simulink model "Furuta_Template"  (Simulink 9.2)
settings: Solver=VariableStepAuto  StartTime=0.0  StopTime=50  FixedStep=0.001  RelTol=1e-8  EnableMultiTasking=on
values from neighbouring files (symbols this model uses):
  A = [0 0 1 0;0 0 0 1;0 LIN1 LIN2 LIN3;0 LIN4 LIN5 LIN6]    [changeable_parameters.m]
  A1 = -J2_hat*b1    (= -5.5028e-07)    [changeable_parameters.m]
  A2 = m2*L1*l2*b2    (= 8.64024e-07)    [changeable_parameters.m]
  A3 = -(J2_hat)^2    (= -3.028080784e-05)    [changeable_parameters.m]
  A4 = -(0.5)*J2_hat*m2*L1*l2    (= -8.49027012e-06)    [changeable_parameters.m]
  A5 = J2_hat*m2*L1*l2    (= 1.698054024e-05)    [changeable_parameters.m]
  A6 = J2_hat    (= 0.0055028)    [changeable_parameters.m]
  A7 = -m2*L1*l2    (= -0.0030858)    [changeable_parameters.m]
  A8 = 0.5*(m2^2)*(l2^2)*L1    (= 1.712619e-05)    [changeable_parameters.m]
  B1 = m2*L1*l2*b1    (= 3.0858e-07)    [changeable_parameters.m]
  B10 = J2_hat    (= 0.0055028)    [changeable_parameters.m]
  B11 = -m2*l2*J0_hat    (= -0.00014201673)    [changeable_parameters.m]
  B12 = -m2*l2*J2_hat    (= -6.108108e-05)    [changeable_parameters.m]
  B2 = -b2*J0_hat    (= -3.582404e-06)    [changeable_parameters.m]
  B3 = -b2*J2_hat    (= -1.540784e-06)    [changeable_parameters.m]
  B4 = m2*L1*l2*J2_hat    (= 1.698054024e-05)    [changeable_parameters.m]
  B5 = 0.5*J0_hat*J2_hat    (= 3.520223702e-05)    [changeable_parameters.m]
  B6 = 0.5*(J2_hat^2)    (= 1.514040392e-05)    [changeable_parameters.m]
  B7 = -0.5*(m2^2)*(L1^2)*(l2^2)    (= -4.76108082e-06)    [changeable_parameters.m]
  B8 = -m2*L1*l2    (= -0.0030858)    [changeable_parameters.m]
  B9 = J0_hat    (= 0.0127943)    [changeable_parameters.m]
  B_mod = [0;0;LIN7;LIN9]    [changeable_parameters.m]
  C = [1 0 0 0 ; 0 1 0 0 ]    [changeable_parameters.m]
  controller_gain_F = - lqr(A,B_mod,Q,R)    [changeable_parameters.m]
  D1 = J0_hat*J2_hat    (= 7.040447404e-05)    [changeable_parameters.m]
  D2 = J2_hat^2    (= 3.028080784e-05)    [changeable_parameters.m]
  D3 = -(m2^2)*(L1^2)*(l2^2)    (= -9.52216164e-06)    [changeable_parameters.m]
  E0 = 0    [changeable_parameters.m]
  G = 9.8    [changeable_parameters.m]
  J2_hat = J2+(m2*(l2^2))    (= 0.0055028)    [changeable_parameters.m]
  K_swingup = 10    [changeable_parameters.m]
  Km = 0.09    [SystemParameters.m]    (also in changeable_parameters.m)
  L = 0.005    [SystemParameters.m]    (also in changeable_parameters.m)
  l2 = 0.148    [SystemParameters.m]    (also in changeable_parameters.m)
  m2 = 0.075    [changeable_parameters.m]
  observer_gain_L = -place (A',C',obs_poles)'    [changeable_parameters.m]
  R = 7.8    [SystemParameters.m]    (also in changeable_parameters.m = B_mod'*Rh*Rh*B_mod)
libraries: simulink x1
settings Model: Creator=mecmg  LastModifiedBy=shady
settings OptimizationCC: ExpressionDepthLimit=2147483647
settings DebuggingCC: SolverPrmCheckMsg=warning

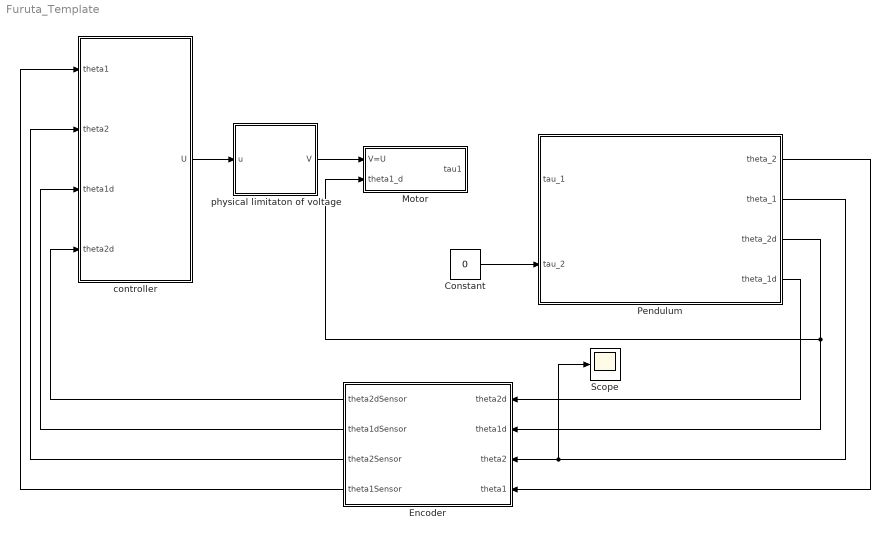
== system Furuta_Template ==
  Constant : Constant  Value=0  VectorParams1D=off
  Encoder : Subsystem
  Motor : Subsystem
  Pendulum : Subsystem
  Scope : Scope
  controller : Subsystem
  physical limitaton of voltage : Subsystem
  wires:
  Pendulum/4(theta_1d) -> Encoder/1(theta2d)
  Pendulum/3(theta_2d) -> Encoder/2(theta1d), Motor/2(theta1_d)
  Pendulum/2(theta_1) -> Scope/1, Encoder/3(theta2)
  Pendulum/1(theta_2) -> Encoder/4(theta1)
  physical limitaton of voltage/1(V) -> Motor/1(V=U)
  Encoder/1(theta2dSensor) -> controller/4(theta2d)
  Encoder/4(theta1Sensor) -> controller/1(theta1)
  Encoder/2(theta1dSensor) -> controller/3(theta1d)
  Encoder/3(theta2Sensor) -> controller/2(theta2)
  Constant/1 -> Pendulum/2(tau_2)
  controller/1("U ") -> physical limitaton of voltage/1(u)

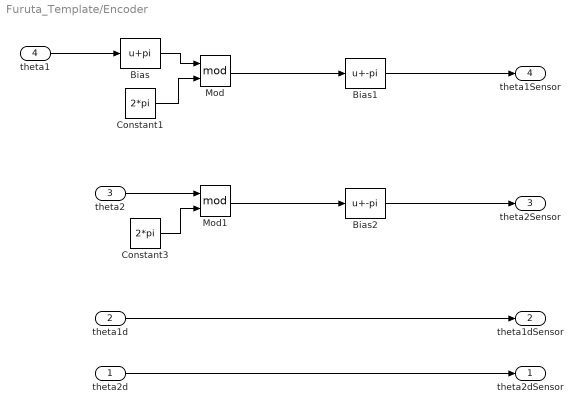
== system Furuta_Template/Encoder ==
  theta2d : Inport
  theta1d : Inport  Port=2
  theta2 : Inport  Port=3
  theta1 : Inport  Port=4
  Bias : Bias  Bias=pi
  Bias1 : Bias  Bias=-pi
  Bias2 : Bias  Bias=-pi
  Constant1 : Constant  Value=2*pi
  Constant3 : Constant  Value=2*pi
  Mod : Math  Operator=mod  SaturateOnIntegerOverflow=on
  Mod1 : Math  Operator=mod  SaturateOnIntegerOverflow=on
  theta2dSensor : Outport
  theta1dSensor : Outport  Port=2
  theta2Sensor : Outport  Port=3
  theta1Sensor : Outport  Port=4
  wires:
  theta1d/1 -> theta1dSensor/1
  theta2d/1 -> theta2dSensor/1
  theta1/1 -> Bias/1
  Constant1/1 -> Mod/2
  theta2/1 -> Mod1/1
  Constant3/1 -> Mod1/2
  Mod1/1 -> Bias2/1
  Bias/1 -> Mod/1
  Mod/1 -> Bias1/1
  Bias1/1 -> theta1Sensor/1
  Bias2/1 -> theta2Sensor/1

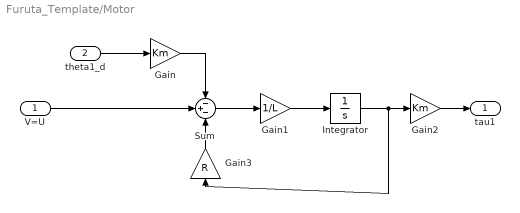
== system Furuta_Template/Motor ==
  V=U : Inport
  theta1_d : Inport  Port=2
  Gain : Gain  Gain=Km
  Gain1 : Gain  Gain=1/L
  Gain2 : Gain  Gain=Km
  Gain3 : Gain  Gain=R
  Integrator : Integrator
  Sum : Sum  Inputs=-+-
  tau1 : Outport
  wires:
  V=U/1 -> Sum/2
  Gain/1 -> Sum/1
  theta1_d/1 -> Gain/1
  Sum/1 -> Gain1/1
  Gain1/1 -> Integrator/1
  Integrator/1 -> Gain3/1, Gain2/1
  Gain2/1 -> tau1/1
  Gain3/1 -> Sum/3

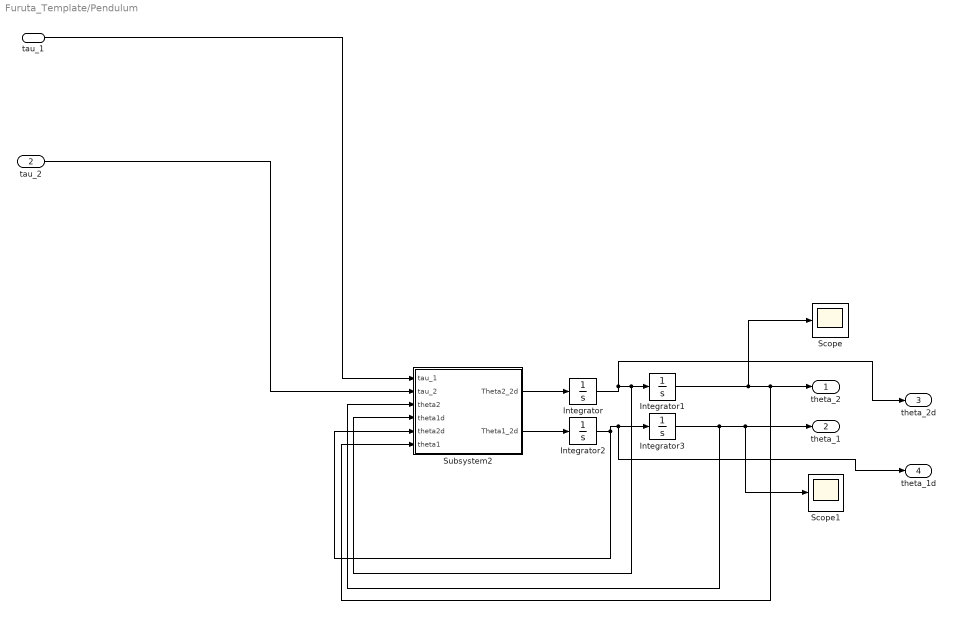
== system Furuta_Template/Pendulum ==
  "tau_1 " : Inport
  tau_2 : Inport  Port=2
  Integrator : Integrator
  Integrator1 : Integrator  InitialCondition=1
  Integrator2 : Integrator
  Integrator3 : Integrator  InitialCondition=1
  Scope : Scope
  Scope1 : Scope
  Subsystem2 : Subsystem
  theta_2 : Outport
  theta_1 : Outport  Port=2
  theta_2d : Outport  Port=3
  theta_1d : Outport  Port=4
  wires:
  tau_2/1 -> Subsystem2/2(tau_2)
  Integrator/1 -> theta_2d/1, Subsystem2/4(theta1d), Integrator1/1
  Integrator3/1 -> Subsystem2/3("theta2 "), Scope1/1, theta_1/1
  Integrator2/1 -> theta_1d/1, Integrator3/1, Subsystem2/5(theta2d)
  "tau_1 "/1 -> Subsystem2/1("tau_1 ")
  Integrator1/1 -> Scope/1, Subsystem2/6(theta1), theta_2/1
  Subsystem2/1(Theta2_2d) -> Integrator/1
  Subsystem2/2(Theta1_2d) -> Integrator2/1

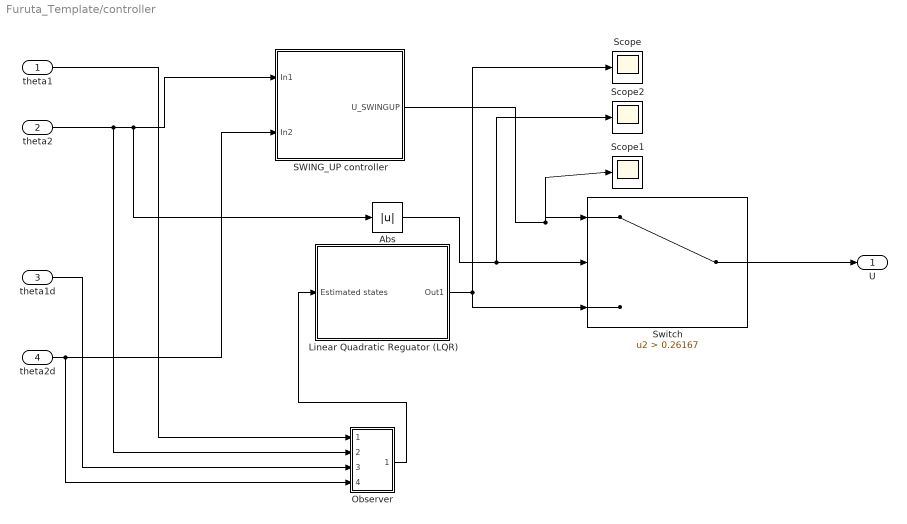
== system Furuta_Template/controller ==
  theta1 : Inport
  theta2 : Inport  Port=2
  theta1d : Inport  Port=3
  theta2d : Inport  Port=4
  " Linear Quadratic Reguator (LQR) " : Subsystem
  " Observer " : Subsystem
  " SWING_UP controller" : Subsystem
  Abs : Abs
  Scope : Scope
  Scope1 : Scope
  Scope2 : Scope
  Switch : Switch  Criteria=u2 > Threshold  Threshold=0.26167
  "U " : Outport
  wires:
  theta2/1 -> " Observer "/2(In3), Abs/1, " SWING_UP controller"/1(In1)
  theta2d/1 -> " Observer "/4(In5), " SWING_UP controller"/2(In2)
  " SWING_UP controller"/1(U_SWINGUP) -> Scope1/1, Switch/1
  Abs/1 -> Scope2/1, Switch/2
  Switch/1 -> "U "/1
  theta1/1 -> " Observer "/1(In1)
  theta1d/1 -> " Observer "/3(In4)
  " Linear Quadratic Reguator (LQR) "/1(Out1) -> Switch/3, Scope/1
  " Observer "/1(Estimated states) -> " Linear Quadratic Reguator (LQR) "/1("Estimated states ")

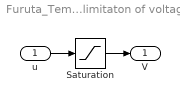
== system Furuta_Template/physical limitaton of voltage ==
  u : Inport
  Saturation : Saturate  UpperLimit=10  LowerLimit=-10
  V : Outport
  wires:
  u/1 -> Saturation/1
  Saturation/1 -> V/1

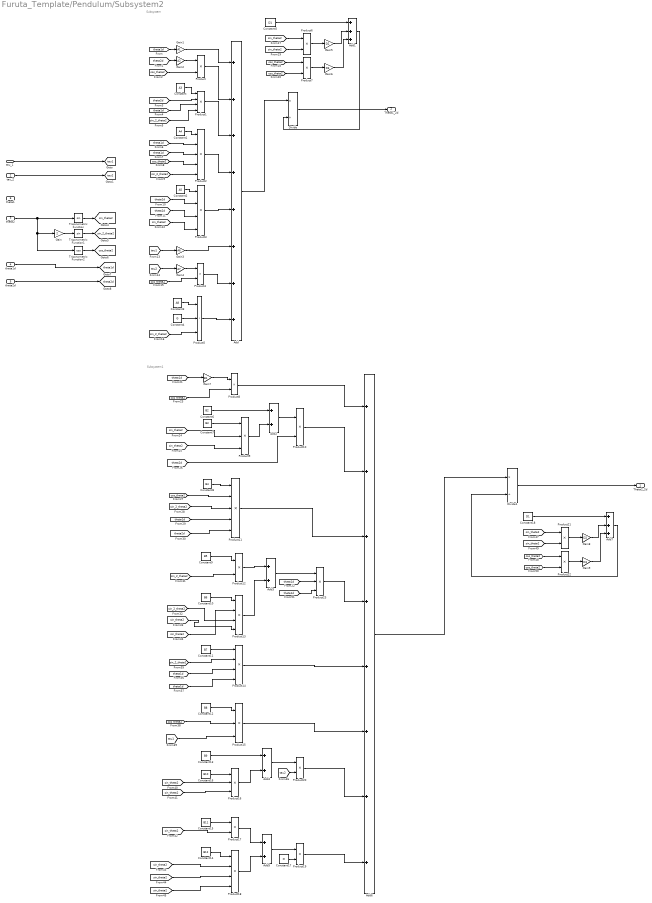
== system Furuta_Template/Pendulum/Subsystem2 ==
  note: Subsystem1
  note: Subsystem
  "tau_1 " : Inport
  tau_2 : Inport  Port=2
  "theta2 " : Inport  Port=3
  theta1d : Inport  Port=4
  theta2d : Inport  Port=5
  theta1 : Inport  Port=6
  Add : Sum  Inputs=8
  Add1 : Sum  Inputs=3
  Add{2..5} (4 alike) : Sum  Inputs=2
  Add6 : Sum  Inputs=8
  Add7 : Sum  Inputs=3
  Constant : Constant  Value=A3  VectorParams1D=off
  Constant1 : Constant  Value=A4  VectorParams1D=off
  Constant10 : Constant  Value=B6
  Constant11 : Constant  Value=B7
  Constant12 : Constant  Value=B8
  Constant13 : Constant  Value=B9
  Constant14 : Constant  Value=B12
  Constant15 : Constant  Value=B11
  Constant16 : Constant  Value=B10
  Constant17 : Constant  Value=G
  Constant18 : Constant  Value=D1
  Constant2 : Constant  Value=A5  VectorParams1D=off
  Constant3 : Constant  Value=A8  VectorParams1D=off
  Constant4 : Constant  Value=G  VectorParams1D=off
  Constant5 : Constant  Value=D1
  Constant6 : Constant  Value=B2
  Constant7 : Constant  Value=B3
  Constant8 : Constant  Value=B4
  Constant9 : Constant  Value=B5
  Divide : Product  Inputs=*/
  Divide1 : Product  Inputs=*/
  Gain : Gain  Gain=2
  Gain1 : Gain  Gain=A1
  Gain2 : Gain  Gain=A2
  Gain3 : Gain  Gain=A6
  Gain4 : Gain  Gain=A7
  Gain5 : Gain  Gain=D2
  Gain6 : Gain  Gain=D3
  Gain7 : Gain  Gain=B1
  Gain8 : Gain  Gain=D2
  Gain9 : Gain  Gain=D3
  Product{,6..7,21..22} (5 alike) : Product  OutMin=2
  Product{1,3,13..14,18} (5 alike) : Product  Inputs=4
  Product{4,8,10,12,17,19..20} (7 alike) : Product
  Product11 : Product  Inputs=5
  Product{5,9,15..16,23} (5 alike) : Product  Inputs=3
  Product2 : Product  Inputs=5
  Trigonometric Function : Trigonometry
  Trigonometric Function1 : Trigonometry
  Trigonometric Function2 : Trigonometry  Operator=cos
  Theta2_2d : Outport
  Theta1_2d : Outport  Port=2
  tag scope: cos_theta2=global, sin_2_theta2=global, sin_theta2=global, tau1=global, tau2=global, theta1d=global, theta2d=global
  wires:
  "theta2 "/1 -> Trigonometric Function2/1, Gain/1, Trigonometric Function/1
  Trigonometric Function1/1 -> [sin_2_theta2]
  theta2d/1 -> [theta2d]
  Trigonometric Function/1 -> [sin_theta2]
  Trigonometric Function2/1 -> [cos_theta2]
  tau_2/1 -> [tau2]
  "tau_1 "/1 -> [tau1]
  theta1d/1 -> [theta1d]
  Gain/1 -> Trigonometric Function1/1
  [theta2d] -> Product1/2
  Gain3/1 -> Add/6
  [sin_theta2] -> Product6/2
  [cos_theta2] -> Product7/2
  [sin_2_theta2] -> Product5/3
  Gain4/1 -> Product4/1
  Add1/1 -> Divide/2
  Product7/1 -> Gain6/1
  Gain1/1 -> Add/1
  [tau2] -> Gain4/1
  Constant1/1 -> Product2/1
  Product6/1 -> Gain5/1
  [cos_theta2] -> Product4/2
  [sin_2_theta2] -> Product2/5
  Product3/1 -> Add/5
  Gain5/1 -> Add1/2
  [theta2d] -> Product3/3
  Constant5/1 -> Add1/1
  [cos_theta2] -> Product7/1
  Gain2/1 -> Product/1
  [theta2d] -> Product3/2
  Product5/1 -> Add/8
  Product1/1 -> Add/3
  Product2/1 -> Add/4
  Gain6/1 -> Add1/3
  [theta1d] -> Product2/3
  [sin_theta2] -> Product3/4
  [cos_theta2] -> Product2/4
  [sin_theta2] -> Product6/1
  [theta1d] -> Product1/3
  Constant/1 -> Product1/1
  [theta1d] -> Product2/2
  [theta2d] -> Gain2/1
  [theta1d] -> Gain1/1
  Add/1 -> Divide/1
  [tau1] -> Gain3/1
  Product4/1 -> Add/7
  Constant4/1 -> Product5/2
  Product/1 -> Add/2
  [cos_theta2] -> Product/2
  Constant2/1 -> Product3/1
  [sin_2_theta2] -> Product1/4
  Constant3/1 -> Product5/1
  Add6/1 -> Divide1/1
  Product12/1 -> Add3/1
  [tau2] -> Product20/2
  [theta2d] -> Product10/2
  Constant9/1 -> Product12/1
  [sin_2_theta2] -> Product14/2
  [tau1] -> Product15/3
  Constant15/1 -> Product17/1
  Constant14/1 -> Product18/1
  [sin_theta2] -> Product16/2
  [sin_theta2] -> Product13/4
  Gain7/1 -> Product8/1
  Product10/1 -> Add6/2
  [theta2d] -> Product11/5
  Constant11/1 -> Product14/1
  Product15/1 -> Add6/6
  [sin_theta2] -> Product16/3
  Product9/1 -> Add2/2
  Product19/1 -> Add6/8
  [sin_theta2] -> Product9/3
  [sin_theta2] -> Product18/2
  Constant17/1 -> Product19/2
  [sin_theta2] -> Product9/2
  Constant6/1 -> Add2/1
  Add2/1 -> Product10/1
  [cos_theta2] -> Product8/2
  Product8/1 -> Add6/1
  [sin_2_theta2] -> Product11/3
  [sin_theta2] -> Product18/3
  Add7/1 -> Divide1/2
  [theta1d] -> Gain7/1
  [cos_theta2] -> Product15/2
  [sin_2_theta2] -> Product13/3
  [cos_theta2] -> Product11/2
  [sin_theta2] -> Product18/4
  Product18/1 -> Add5/2
  Constant8/1 -> Product11/1
  Product20/1 -> Add6/7
  Add5/1 -> Product19/1
  [sin_theta2] -> Product21/2
  Constant10/1 -> Product13/1
  Constant12/1 -> Product15/1
  Product22/1 -> Gain9/1
  Product16/1 -> Add4/2
  Product13/1 -> Add3/2
  Product21/1 -> Gain8/1
  Constant16/1 -> Product16/1
  Constant7/1 -> Product9/1
  Product17/1 -> Add5/1
  Constant18/1 -> Add7/1
  Constant13/1 -> Add4/1
  [cos_theta2] -> Product22/1
  Gain9/1 -> Add7/3
  [cos_theta2] -> Product22/2
  [sin_theta2] -> Product21/1
  [theta1d] -> Product11/4
  Product14/1 -> Add6/5
  Product11/1 -> Add6/3
  [sin_theta2] -> Product17/2
  Gain8/1 -> Add7/2
  Add4/1 -> Product20/1
  Divide1/1 -> Theta2_2d/1
  Divide/1 -> Theta1_2d/1
  Add3/1 -> Product23/1
  [theta1d] -> Product23/2
  [theta1d] -> Product23/3
  [sin_2_theta2] -> Product12/2
  [sin_theta2] -> Product13/2
  Product23/1 -> Add6/4
  [theta1d] -> Product14/3
  [theta1d] -> Product14/4

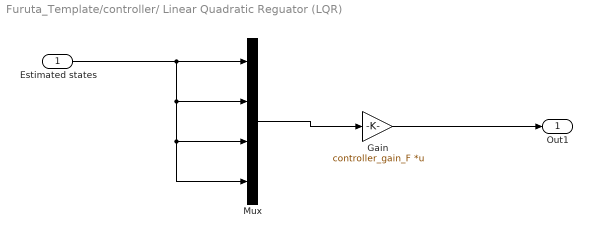
== system Furuta_Template/controller/ Linear Quadratic Reguator (LQR)  ==
  "Estimated states " : Inport
  Gain : Gain  Gain=controller_gain_F  Multiplication=Matrix(K*u)
  Mux : Mux
  Out1 : Outport
  wires:
  Mux/1 -> Gain/1
  Gain/1 -> Out1/1
  "Estimated states "/1 -> Mux/4, Mux/3, Mux/2, Mux/1

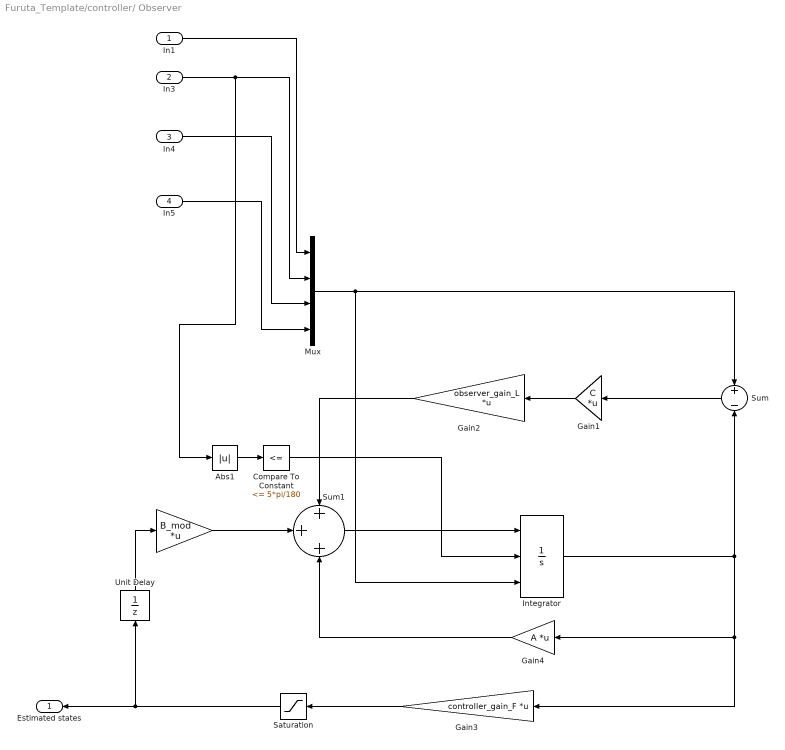
== system Furuta_Template/controller/ Observer  ==
  In1 : Inport
  In3 : Inport  Port=2
  In4 : Inport  Port=3
  In5 : Inport  Port=4
  " " : Gain  Gain=B_mod  Multiplication=Matrix(K*u)
  Abs1 : Abs
  Compare To Constant : simulink/Logic and Bit Operations/Compare To Constant  relop=<=  const=5*pi/180  OutDataTypeStr=boolean
  Gain1 : Gain  Gain=C  Multiplication=Matrix(K*u)
  Gain2 : Gain  Gain=observer_gain_L  Multiplication=Matrix(K*u)
  Gain3 : Gain  Gain=controller_gain_F  Multiplication=Matrix(K*u)
  Gain4 : Gain  Gain=A  Multiplication=Matrix(K*u)
  Integrator : Integrator  ExternalReset=rising  InitialConditionSource=external  LimitOutput=on  UpperSaturationLimit=25000  LowerSaturationLimit=-25000  ZeroCross=off
  Mux : Mux
  Saturation : Saturate
  Sum : Sum  Inputs=+-
  Sum1 : Sum  Inputs=+++
  Unit Delay : UnitDelay  SampleTime=-1
  Estimated states : Outport
  wires:
  In1/1 -> Mux/1
  Gain4/1 -> Sum1/3
  Integrator/1 -> Sum/2, Gain3/1, Gain4/1
  " "/1 -> Sum1/2
  Mux/1 -> Integrator/3, Sum/1
  Gain2/1 -> Sum1/1
  Unit Delay/1 -> " "/1
  Sum/1 -> Gain1/1
  Compare To Constant/1 -> Integrator/2
  Saturation/1 -> Unit Delay/1, Estimated states/1
  Gain3/1 -> Saturation/1
  Abs1/1 -> Compare To Constant/1
  In3/1 -> Mux/2, Abs1/1
  In5/1 -> Mux/4
  In4/1 -> Mux/3
  Gain1/1 -> Gain2/1
  Sum1/1 -> Integrator/1

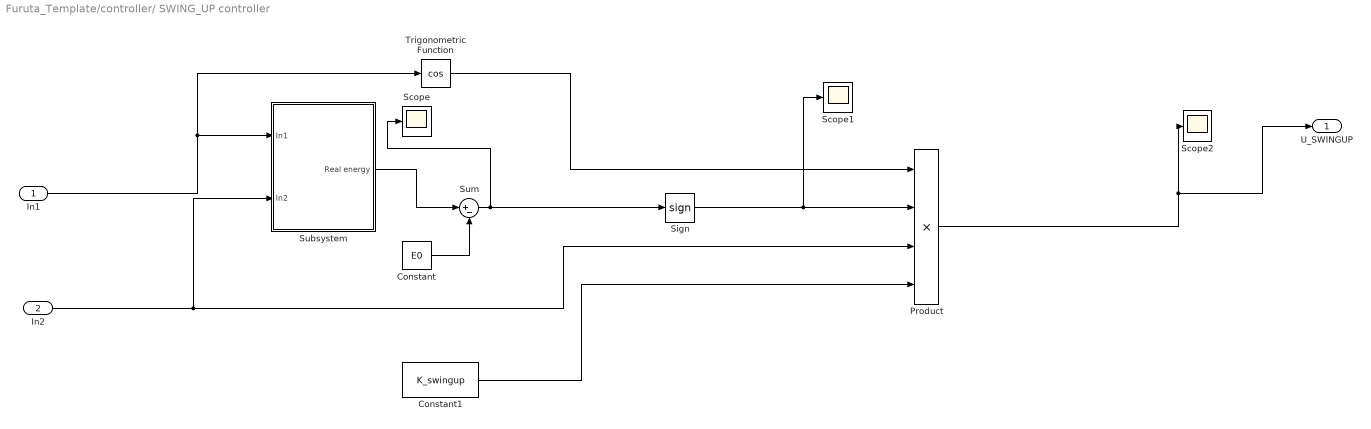
== system Furuta_Template/controller/ SWING_UP controller ==
  In1 : Inport
  In2 : Inport  Port=2
  Constant : Constant  Value=E0
  Constant1 : Constant  Value=K_swingup
  Product : Product  Inputs=4
  Scope : Scope
  Scope1 : Scope
  Scope2 : Scope
  Sign : Signum
  Subsystem : Subsystem
  Sum : Sum  Inputs=|+-
  Trigonometric Function : Trigonometry  Operator=cos
  U_SWINGUP : Outport
  wires:
  Subsystem/1("Real energy ") -> Sum/1
  In1/1 -> Trigonometric Function/1, Subsystem/1(In1)
  Sign/1 -> Scope1/1, Product/2
  Constant1/1 -> Product/4
  Sum/1 -> Scope/1, Sign/1
  Trigonometric Function/1 -> Product/1
  In2/1 -> Subsystem/2(In2), Product/3
  Product/1 -> U_SWINGUP/1, Scope2/1
  Constant/1 -> Sum/2

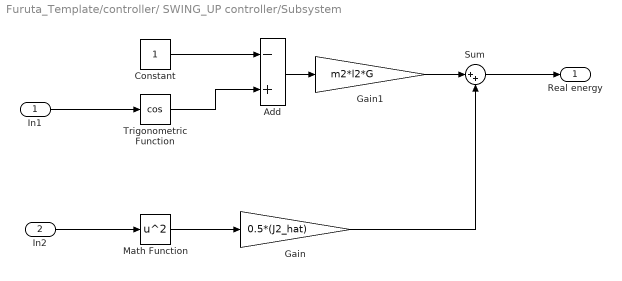
== system Furuta_Template/controller/ SWING_UP controller/Subsystem ==
  In1 : Inport
  In2 : Inport  Port=2
  Add : Sum  Inputs=-+
  Constant : Constant
  Gain : Gain  Gain=0.5*(J2_hat)
  Gain1 : Gain  Gain=m2*l2*G
  Math Function : Math  Operator=square  SaturateOnIntegerOverflow=on
  Sum : Sum  Inputs=|++
  Trigonometric Function : Trigonometry  Operator=cos
  "Real energy " : Outport
  wires:
  Math Function/1 -> Gain/1
  In1/1 -> Trigonometric Function/1
  Gain1/1 -> Sum/1
  Gain/1 -> Sum/2
  Constant/1 -> Add/1
  Trigonometric Function/1 -> Add/2
  In2/1 -> Math Function/1
  Add/1 -> Gain1/1
  Sum/1 -> "Real energy "/1
